simulink model "armModelLQG"  (R2018b)
settings: Solver=ode15s  StartTime=0.0  StopTime=10  MaxStep=1e-4  RelTol=1e-6  AbsTol=1e-7
values from neighbouring files (symbols this model uses):
  Cv1 = 1.3*10^(-6)*60/(2*pi)    (= 1.24140855612e-05)    [setup.m]
  Cv2 = 1.3*10^(-6)*60/(2*pi)    (= 1.24140855612e-05)    [setup.m]
  Cv3 = 1.3*10^(-6)*60/(2*pi)    (= 1.24140855612e-05)    [setup.m]
  effWorm = 0.8    [setup.m]
  J1 = 1.3*10^(-4)    (= 0.00013)    [setup.m]
  J2 = 0.79*10^(-4)    (= 7.9e-05)    [setup.m]
  J3 = 0.98*10^(-4)    (= 9.8e-05)    [setup.m]
  Ke1 = 0.15    [setup.m]
  Ke2 = 0.12    [setup.m]
  Ke3 = 0.12    [setup.m]
  Km1 = 0.15    [setup.m]
  Km2 = 0.12    [setup.m]
  Km3 = 0.12    [setup.m]
  N1 = 36    [setup.m]
  N2 = 36    [setup.m]
  N3 = 36    [setup.m]
  R1 = 1.9    [setup.m]
  R2 = 2.45    [setup.m]
  R3 = 1.9    [setup.m]
undefined symbols (not defined in the file or in its folder): A, B, C, Continuous, D, Time, X, Y, Z
libraries: sm_lib x92, nesl_utility x26, simulink x5, Parts_Lib x2, Contact_Forces_Lib x2, ctrlSharedLib x1
(part 1 of 4)
settings Model: Creator=jurp1  LastModifiedBy=Dennis
settings DataIOCC: SaveState=on
settings DebuggingCC: LibraryContextMissingDiagnostic=none  UnderSpecifiedDimensionMsg=warning
settings SFSimCC: SimUseLocalCustomCode=off
settings RTWCC: RTWUseLocalCustomCode=off

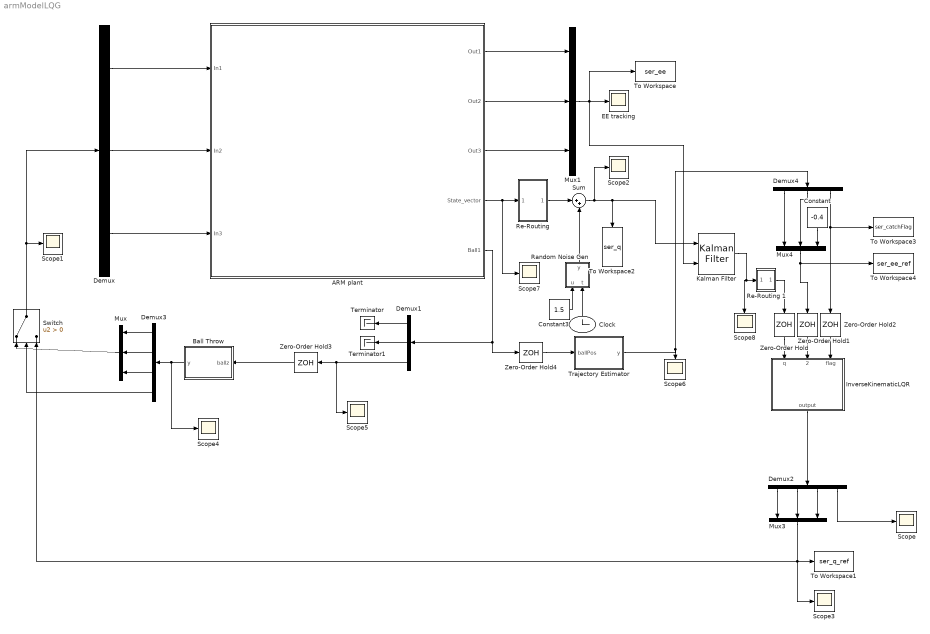
== system armModelLQG ==
  "ARM plant " : Subsystem
  Ball Throw : MATLAB Function  TreatAsAtomicUnit=on
  Clock : Clock
  Constant : Constant  Value=-0.4
  Constant3 : Constant  Value=1.5
  Demux : Demux  Outputs=3
  Demux1 : Demux  Outputs=3
  Demux2 : Demux
  Demux3 : Demux
  Demux4 : Demux  Outputs=3
  EE tracking : Scope
  "InverseKinematicLQR " : MATLAB Function  TreatAsAtomicUnit=on
  Kalman Filter : ctrlSharedLib/Kalman Filter  TimeDomain=Continuous-Time  UseCurrentEstimator=on  ModelSource=Individual A, B, C, D matrices  ModelSourceVariable=ss(0.95,1,1,0,1)  A=A  B=B  C=C  D=D  NumberOfStates=1  NumberOfInputs=1  NumberOfOutputs=1  InitialEstimateSource=Dialog  X0=0  P0=10  UseK=off  UseGH=off  NumberOfProcessNoiseInputs=1  G=1  TimeInvariantG=on  H=0  TimeInvariantH=on  Q=0.05  TimeInvariantQ=on  R=1  TimeInvariantR=on  N=0  TimeInvariantN=on  AddInputPort=on  AddEnablePort=off  OutputEstimatedY=off  OutputP=off  Ts=-1
      settings: SourceProductBaseCode=CT
  Mux{,1,3..4} (4 alike) : Mux  Inputs=3
  Random Noise Gen : MATLAB Function  TreatAsAtomicUnit=on
  "Re-Routing " : Subsystem
  Re-Routing 1 : Subsystem
  Scope{,1..8} (9 alike) : Scope
  Sum : Sum  Inputs=|++
  Switch : Switch  Criteria=u2 > Threshold
  Terminator : Terminator
  Terminator1 : Terminator
  To Workspace : ToWorkspace  VariableName=ser_ee  SaveFormat=Timeseries  SampleTime=0.0001
  To Workspace1 : ToWorkspace  VariableName=ser_q_ref  SaveFormat=Timeseries  SampleTime=0.0001
  To Workspace2 : ToWorkspace  VariableName=ser_q  SaveFormat=Timeseries  SampleTime=0.0001
  To Workspace3 : ToWorkspace  VariableName=ser_catchFlag  SaveFormat=Timeseries  SampleTime=-1
  To Workspace4 : ToWorkspace  VariableName=ser_ee_ref  SaveFormat=Timeseries  SampleTime=0.0001
  Trajectory Estimator : MATLAB Function  TreatAsAtomicUnit=on
  Zero-Order Hold : ZeroOrderHold  SampleTime=0.001
  Zero-Order Hold1 : ZeroOrderHold  SampleTime=0.001
  Zero-Order Hold2 : ZeroOrderHold  SampleTime=0.001
  Zero-Order Hold3 : ZeroOrderHold  SampleTime=0.1
  Zero-Order Hold4 : ZeroOrderHold  SampleTime=0.01
  wires:
  "ARM plant "/1(Out1) -> Mux1/1
  "ARM plant "/2(Out2) -> Mux1/2
  "ARM plant "/3(Out3) -> Mux1/3
  Demux/1 -> "ARM plant "/1(In1)
  Demux/2 -> "ARM plant "/2(In2)
  Demux/3 -> "ARM plant "/3(In3)
  "ARM plant "/4("State_vector ") -> Scope7/1, "Re-Routing "/1(In1)
  "InverseKinematicLQR "/1(output) -> Demux2/1
  Zero-Order Hold2/1 -> "InverseKinematicLQR "/3(flag)
  Zero-Order Hold1/1 -> "InverseKinematicLQR "/2(state_trgt)
  Zero-Order Hold/1 -> "InverseKinematicLQR "/1(q)
  Demux2/2 -> Mux3/2
  Demux2/3 -> Mux3/3
  Demux2/1 -> Mux3/1
  Mux3/1 -> Switch/3, To Workspace1/1, Scope3/1
  Demux2/4 -> Scope/1
  Switch/1 -> Scope1/1, Demux/1
  "ARM plant "/5(Ball1) -> Zero-Order Hold4/1, Demux1/1
  Demux1/3 -> Scope5/1, Zero-Order Hold3/1
  Zero-Order Hold3/1 -> Ball Throw/1(ballz)
  Ball Throw/1(y) -> Scope4/1, Demux3/1
  Demux3/2 -> Mux/2
  Demux3/1 -> Mux/1
  Demux3/3 -> Mux/3
  Demux3/4 -> Switch/2
  Mux/1 -> Switch/1
  Demux1/2 -> Terminator1/1
  Demux1/1 -> Terminator/1
  Zero-Order Hold4/1 -> Trajectory Estimator/1(ballPos)
  Trajectory Estimator/1(y) -> Demux4/1, Scope6/1
  Demux4/3 -> Zero-Order Hold2/1, To Workspace3/1
  Constant/1 -> Mux4/3
  Demux4/2 -> Mux4/2
  Demux4/1 -> Mux4/1
  Mux4/1 -> Zero-Order Hold1/1, To Workspace4/1
  Constant3/1 -> Random Noise Gen/1(u)
  Random Noise Gen/1(y) -> Sum/2
  "Re-Routing "/1(Out1) -> Sum/1
  Clock/1 -> Random Noise Gen/2(t)
  Kalman Filter/1 -> Scope8/1, Re-Routing 1/1(In1)
  Sum/1 -> Scope2/1, To Workspace2/1, Kalman Filter/1
  Re-Routing 1/1(Out1) -> Zero-Order Hold/1
  Mux1/1 -> Kalman Filter/2, To Workspace/1, EE tracking/1
